simulink model "sampleModel1674_5_sub"  (R2023a)
settings: Solver=VariableStepAuto  StartTime=0.0  StopTime=10.0  RelTol=1e-3
libraries: hdlsllib x6, simulink x4
settings Model: Creator=user1  LastModifiedBy=user1

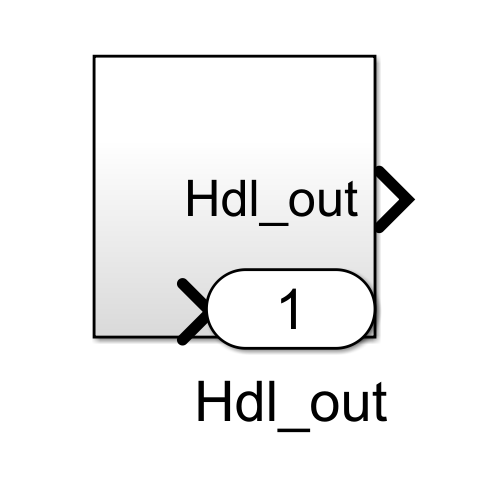
[thumbnail: Simulink's stored preview of the top-level diagram]
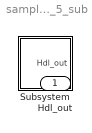
== system sampleModel1674_5_sub ==
  Subsystem : Subsystem
  Hdl_out : Outport  OutDataTypeStr=uint8

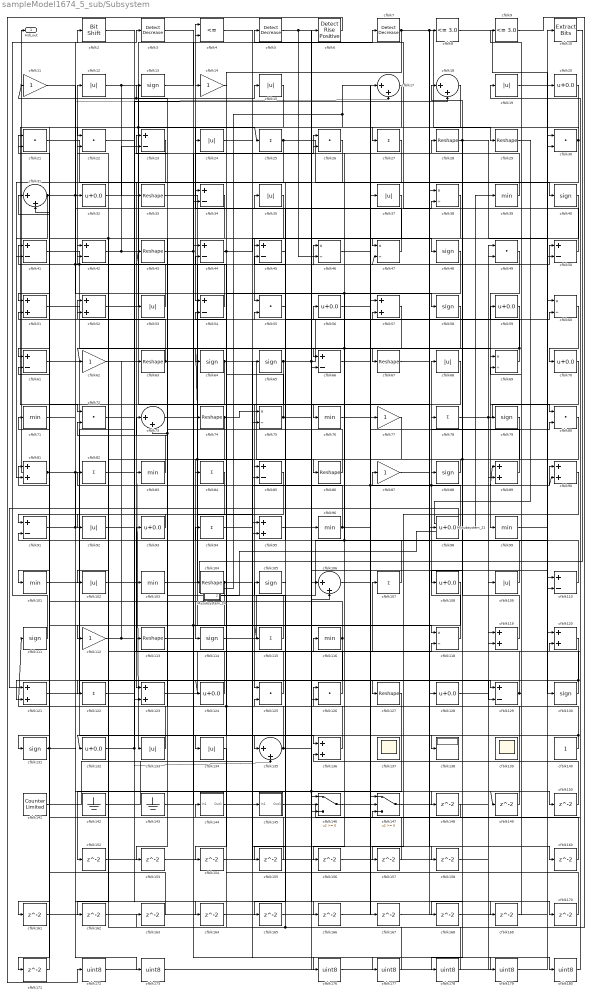
== system sampleModel1674_5_sub/Subsystem ==
  Mysubsystem_21 : Subsystem  TreatAsAtomicUnit=on  RTWFcnName=Mysubsystem_21
      settings: RTWFcnNameOpts=User specified  RTWFileNameOpts=Use function name
  Mysubsystem_24 : Subsystem  TreatAsAtomicUnit=on  RTWFcnName=Mysubsystem_24
      settings: RTWFcnNameOpts=User specified  RTWFileNameOpts=Use function name
  cfblk10 : simulink/Logic and Bit Operations/Extract Bits  bitsToExtract=Upper half  numBits=8  bitIdxRange=[0 7]  outScalingMode=Preserve fixed-point scaling
      settings: LibrarySourceBlock=|
      | hdlsllib/Logic and Bit
      | Operations/Extract Bits
  cfblk{39,71,76,83,96,99,101,103,116} (9 alike) : MinMax  OutDataTypeStr=uint8
  cfblk{12,15,19,24,35,37,53,68,92,102,109,133..134} (13 alike) : Abs  OutDataTypeStr=uint8  SaturateOnIntegerOverflow=off
  cfblk{28..29,33,43,63,67,74,86,104,113,127} (11 alike) : Reshape
  cfblk{13,40,48,58,64..65,79,88,105,111,114,130..131} (13 alike) : Signum
  cfblk{17..18,31,73,106,135} (6 alike) : Sum  Inputs=|++  OutDataTypeStr=uint8
  cfblk{25,27,78,82,84,94,107,115,122} (9 alike) : Sum  Inputs=+  OutDataTypeStr=uint8
  cfblk{20,32,56,59,70,93,98,108,124,128,132} (11 alike) : Bias  Bias=0.0  SaturateOnIntegerOverflow=off
  cfblk{11,14,62,77,87,112} (6 alike) : Gain  OutDataTypeStr=uint8
  cfblk{23,34,41..42,44..45,50,54,61,66,85,91,110,129} (14 alike) : Sum  Inputs=+-  OutDataTypeStr=uint8
  cfblk{38,46..47,60,69,75,118} (7 alike) : Product  Inputs=*/  OutDataTypeStr=uint8  RndMeth=Zero  SaturateOnIntegerOverflow=on
  cfblk{51..52,57,81,89..90,95,119..121,123,136} (12 alike) : Sum  OutDataTypeStr=uint8
  cfblk{21..22,26,30,49,55,72,80,125..126} (10 alike) : DotProduct  OutDataTypeStr=uint8
  cfblk137 : Scope
      settings: Floating=on
  cfblk138 : Display
  cfblk139 : Scope
      settings: Floating=on
  cfblk140 : Constant  OutDataTypeStr=uint8  SampleTime=-1
  cfblk141 : hdlsllib/Sources/Counter Limited  uplimit=7  tsamp=-1
  cfblk142 : Ground
  cfblk143 : Ground
  cfblk144 : Subsystem
      settings: LibrarySourceBlock=|
      | hdlsllib/Ports &
      | Subsystems/Subsystem
  cfblk145 : Subsystem
      settings: LibrarySourceBlock=|
      | hdlsllib/Ports &
      | Subsystems/Subsystem
  cfblk146 : Switch  OutDataTypeStr=uint8  SaturateOnIntegerOverflow=off  InputSameDT=off
  cfblk147 : Switch  OutDataTypeStr=uint8  SaturateOnIntegerOverflow=off  InputSameDT=off
  cfblk{148..150,152..158,160..171} (22 alike) : Delay  SampleTime=1
  cfblk{172..173,176..180} (7 alike) : DataTypeConversion  OutDataTypeStr=uint8  SaturateOnIntegerOverflow=off  RndMeth=Floor
  cfblk2 : hdlsllib/Logic and Bit Operations/Bit Shift  mode=Shift Left Logical  N=0
  cfblk3 : simulink/Logic and Bit Operations/Detect Decrease  vinit=0.0  OutDataTypeStr=uint8
      settings: LibrarySourceBlock=|
      | hdlsllib/Logic and Bit
      | Operations/Detect
      | Decrease
  cfblk4 : RelationalOperator  Operator=<=  OutDataTypeStr=boolean  InputSameDT=off
  cfblk5 : simulink/Logic and Bit Operations/Detect Decrease  vinit=0.0  OutDataTypeStr=uint8
      settings: LibrarySourceBlock=|
      | hdlsllib/Logic and Bit
      | Operations/Detect
      | Decrease
  cfblk6 : hdlsllib/Logic and Bit Operations/Detect Rise Positive  vinit=0  OutDataTypeStr=uint8
  cfblk7 : simulink/Logic and Bit Operations/Detect Decrease  vinit=0.0  OutDataTypeStr=uint8
      settings: LibrarySourceBlock=|
      | hdlsllib/Logic and Bit
      | Operations/Detect
      | Decrease
  cfblk8 : hdlsllib/Logic and Bit Operations/Compare To Constant  relop=<=  const=3.0  OutDataTypeStr=uint8
  cfblk9 : hdlsllib/Logic and Bit Operations/Compare To Constant  relop=<=  const=3.0  OutDataTypeStr=uint8
  Hdl_out : Outport  OutDataTypeStr=uint8
  wires:
  cfblk98/1 -> cfblk39/1, cfblk87/1
  cfblk34/1 -> cfblk162/1, cfblk161/1
  cfblk61/1 -> cfblk136/1
  cfblk7/1 -> cfblk34/1, cfblk160/1, cfblk29/1
  cfblk17/1 -> cfblk72/1
  cfblk50/1 -> cfblk5/1
  cfblk140/1 -> cfblk132/1, cfblk126/1
  cfblk43/1 -> cfblk179/1, cfblk26/2
  cfblk68/1 -> cfblk125/1
  cfblk74/1 -> cfblk75/1, cfblk114/1
  cfblk35/1 -> cfblk55/1
  cfblk101/1 -> cfblk129/1
  cfblk51/1 -> cfblk55/2
  cfblk120/1 -> cfblk178/1
  cfblk93/1 -> cfblk91/1
  cfblk3/1 -> cfblk177/1, cfblk115/1
  cfblk53/1 -> cfblk12/1
  cfblk30/1 -> cfblk27/1, cfblk85/1
  cfblk15/1 -> cfblk51/1
  cfblk79/1 -> cfblk168/1, cfblk133/1
  cfblk41/1 -> cfblk43/1, cfblk67/1
  cfblk145/1(Out1) -> cfblk19/1
  cfblk33/1 -> cfblk118/1
  cfblk71/1 -> cfblk17/2, cfblk32/1
  cfblk88/1 -> cfblk86/1
  cfblk125/1 -> cfblk42/1
  cfblk27/1 -> cfblk123/1
  cfblk11/1 -> cfblk58/1
  cfblk131/1 -> cfblk169/1, cfblk41/1
  cfblk94/1 -> cfblk149/1, cfblk146/3
  cfblk128/1 -> cfblk119/1
  cfblk64/1 -> cfblk101/1, cfblk96/1
  cfblk39/1 -> cfblk4/1
  cfblk67/1 -> cfblk8/1
  cfblk69/1 -> cfblk45/2, cfblk62/1
  cfblk47/1 -> cfblk14/1
  cfblk20/1 -> cfblk22/1
  cfblk42/1 -> cfblk23/2, cfblk4/2
  cfblk14/1 -> cfblk134/1
  cfblk65/1 -> cfblk113/1, cfblk110/2, cfblk57/2
  cfblk121/1 -> cfblk56/1
  cfblk126/1 -> cfblk93/1
  cfblk123/1 -> cfblk65/1
  cfblk8/1 -> cfblk110/1
  cfblk38/1 -> cfblk83/1, cfblk73/2
  cfblk76/1 -> cfblk17/1
  cfblk118/1 -> cfblk68/1
  cfblk83/1 -> cfblk72/2
  cfblk103/1 -> cfblk46/1
  cfblk73/1 -> cfblk145/1(In1), cfblk95/2
  cfblk129/1 -> cfblk82/1, cfblk9/1
  cfblk78/1 -> cfblk60/2, cfblk80/1
  cfblk119/1 -> cfblk18/1
  cfblk32/1 -> cfblk66/1
  cfblk85/1 -> cfblk123/2
  cfblk23/1 -> cfblk41/2
  cfblk12/1 -> cfblk33/1, cfblk25/1, cfblk147/2
  cfblk58/1 -> cfblk92/1
  cfblk4/1 -> cfblk48/1
  cfblk52/1 -> cfblk15/1
  cfblk107/1 -> cfblk26/1, cfblk81/1
  cfblk54/1 -> cfblk21/1
  cfblk111/1 -> cfblk2/1
  cfblk57/1 -> cfblk74/1, cfblk76/1
  cfblk136/1 -> cfblk94/1, cfblk111/1
  cfblk18/1 -> cfblk54/1
  cfblk87/1 -> cfblk128/1
  cfblk44/1 -> cfblk47/1, cfblk84/1
  cfblk25/1 -> cfblk40/1, cfblk131/1
  cfblk31/1 -> cfblk3/1, cfblk81/2
  cfblk60/1 -> cfblk70/1
  cfblk96/1 -> cfblk52/1, cfblk88/1, cfblk90/2
  cfblk112/1 -> cfblk63/1, cfblk53/1
  cfblk70/1 -> cfblk99/1
  cfblk130/1 -> cfblk124/1, cfblk107/1
  cfblk21/1 -> cfblk126/2
  cfblk147/1 -> cfblk49/1
  cfblk13/1 -> cfblk7/1
  cfblk114/1 -> cfblk10/1
  cfblk106/1 -> cfblk37/1
  cfblk116/1 -> cfblk51/2, cfblk121/2
  cfblk2/1 -> cfblk103/1
  cfblk46/1 -> cfblk77/1
  cfblk81/1 -> Hdl_out/1, cfblk146/2, cfblk50/1
  cfblk63/1 -> cfblk75/2, cfblk31/2
  cfblk89/1 -> cfblk78/1
  cfblk115/1 -> cfblk23/1
  cfblk99/1 -> cfblk30/2
  cfblk92/1 -> cfblk24/1
  cfblk40/1 -> cfblk61/1
  cfblk146/1 -> cfblk80/2, cfblk89/1
  cfblk75/1 -> cfblk44/2, cfblk127/1
  cfblk19/1 -> cfblk130/1
  cfblk141/1 -> cfblk44/1
  cfblk143/1 -> cfblk104/1
  cfblk49/1 -> cfblk79/1
  cfblk132/1 -> cfblk135/2, cfblk116/1
  cfblk109/1 -> cfblk28/1
  cfblk135/1 -> cfblk71/1, cfblk59/1
  cfblk91/1 -> cfblk173/1, cfblk47/2, cfblk38/2
  cfblk77/1 -> cfblk102/1
  cfblk86/1 -> cfblk13/1, cfblk11/1
  cfblk59/1 -> cfblk66/2
  cfblk104/1 -> cfblk180/1, cfblk122/1
  cfblk122/1 -> cfblk18/2
  cfblk95/1 -> cfblk106/2
  cfblk62/1 -> cfblk98/1
  cfblk124/1 -> cfblk52/2
  cfblk56/1 -> cfblk69/1
  cfblk37/1 -> cfblk112/1
  cfblk110/1 -> cfblk35/1
  cfblk5/1 -> cfblk170/1, cfblk46/2
  cfblk133/1 -> cfblk61/2
  cfblk28/1 -> cfblk50/2, cfblk108/1
  cfblk45/1 -> cfblk135/1
  cfblk113/1 -> cfblk118/2
  cfblk80/1 -> cfblk138/1
  cfblk48/1 -> cfblk156/1, cfblk64/1
  cfblk142/1 -> cfblk90/1
  cfblk26/1 -> cfblk45/1
  cfblk102/1 -> cfblk148/1
  cfblk148/1 -> cfblk147/3
  cfblk149/1 -> cfblk73/1
  cfblk72/1 -> cfblk150/1
  cfblk150/1 -> cfblk136/2
  cfblk127/1 -> cfblk152/1
  cfblk152/1 -> cfblk95/1
  cfblk84/1 -> cfblk153/1
  cfblk153/1 -> cfblk57/1
  cfblk134/1 -> cfblk154/1
  cfblk154/1 -> cfblk85/2
  cfblk55/1 -> cfblk155/1
  cfblk155/1 -> cfblk21/2
  cfblk156/1 -> cfblk49/2
  cfblk90/1 -> cfblk157/1
  cfblk157/1 -> cfblk125/2
  cfblk24/1 -> cfblk158/1
  cfblk158/1 -> cfblk89/2
  cfblk160/1 -> cfblk42/2
  cfblk161/1 -> cfblk147/1
  cfblk162/1 -> cfblk146/1
  cfblk9/1 -> cfblk163/1
  cfblk163/1 -> cfblk91/2
  cfblk82/1 -> cfblk164/1
  cfblk164/1 -> cfblk30/1
  cfblk105/1 -> cfblk165/1
  cfblk165/1 -> cfblk106/1
  cfblk22/1 -> cfblk166/1
  cfblk166/1 -> cfblk60/1
  cfblk66/1 -> cfblk167/1
  cfblk167/1 -> cfblk38/1
  cfblk168/1 -> cfblk119/2
  cfblk169/1 -> cfblk69/2
  cfblk170/1 -> cfblk54/2
  cfblk108/1 -> cfblk171/1
  cfblk171/1 -> cfblk31/1
  cfblk6/1 -> cfblk172/1
  cfblk172/1 -> cfblk20/1
  cfblk173/1 -> cfblk6/1
  cfblk144/1(Out1) -> cfblk176/1
  cfblk176/1 -> cfblk109/1
  cfblk177/1 -> cfblk144/1(In1)
  cfblk178/1 -> cfblk105/1, cfblk22/2
  cfblk179/1 -> cfblk120/1
  cfblk180/1 -> cfblk120/2
  cfblk29/1 -> Mysubsystem_21/1(In1)
  Mysubsystem_21/1(Out1) -> cfblk121/1
  Mysubsystem_24/1(Out1) -> cfblk34/2, cfblk129/2
  cfblk10/1 -> Mysubsystem_24/1(In1)
  Mysubsystem_24/2(Out2) -> Mysubsystem_21/2(In2)

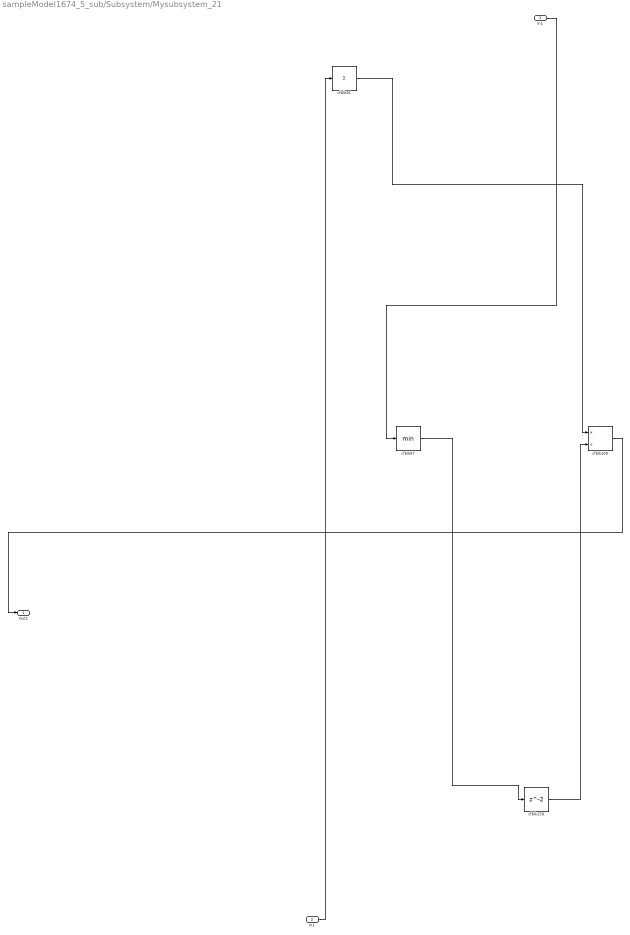
== system sampleModel1674_5_sub/Subsystem/Mysubsystem_21 ==
  In1 : Inport
  In2 : Inport  Port=2
  cfblk100 : Product  Inputs=*/  RndMeth=Zero  SaturateOnIntegerOverflow=on
  cfblk159 : Delay  SampleTime=1
  cfblk36 : Sum  Inputs=+
  cfblk97 : MinMax
  Out1 : Outport
  wires:
  In1/1 -> cfblk97/1
  cfblk100/1 -> Out1/1
  In2/1 -> cfblk36/1
  cfblk159/1 -> cfblk100/2
  cfblk36/1 -> cfblk100/1
  cfblk97/1 -> cfblk159/1

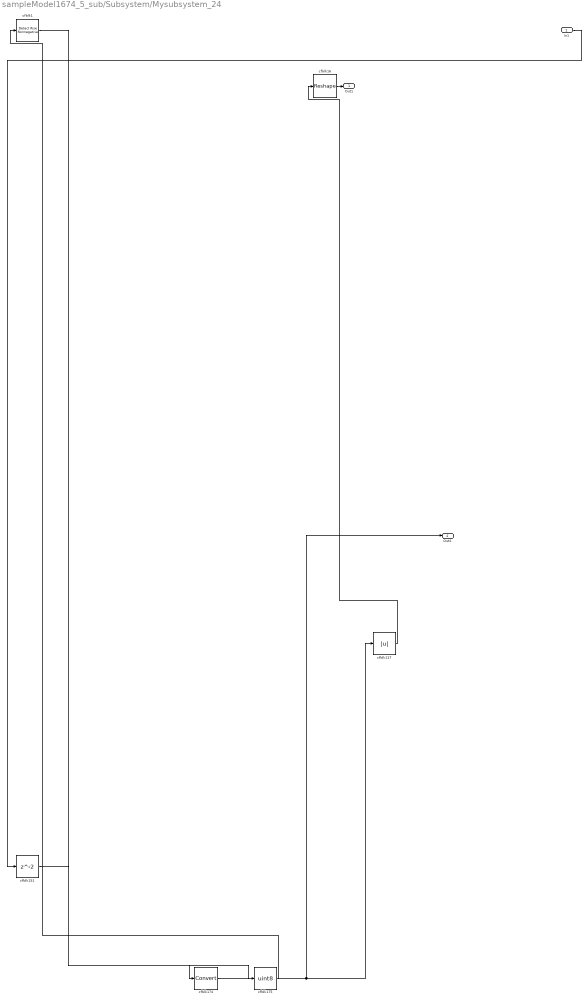
== system sampleModel1674_5_sub/Subsystem/Mysubsystem_24 ==
  In1 : Inport
  cfblk1 : hdlsllib/Logic and Bit Operations/Detect Rise Nonnegative  vinit=0  OutDataTypeStr=boolean
  cfblk117 : Abs  SaturateOnIntegerOverflow=off
  cfblk151 : Delay  SampleTime=1
  cfblk16 : Reshape
  cfblk174 : DataTypeConversion  SaturateOnIntegerOverflow=off  RndMeth=Floor
  cfblk175 : DataTypeConversion  OutDataTypeStr=uint8  SaturateOnIntegerOverflow=off  RndMeth=Floor
  Out1 : Outport
  Out2 : Outport  Port=2
  wires:
  cfblk151/1 -> cfblk175/1
  In1/1 -> cfblk151/1
  cfblk117/1 -> cfblk16/1
  cfblk1/1 -> cfblk174/1
  cfblk175/1 -> cfblk1/1
  cfblk16/1 -> Out1/1
  cfblk174/1 -> cfblk117/1, Out2/1

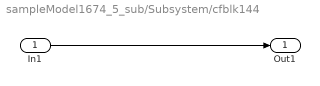
== system sampleModel1674_5_sub/Subsystem/cfblk144 ==
  In1 : Inport
  Out1 : Outport
  wires:
  In1/1 -> Out1/1

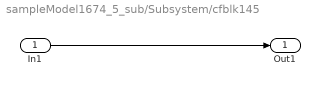
== system sampleModel1674_5_sub/Subsystem/cfblk145 ==
  In1 : Inport
  Out1 : Outport
  wires:
  In1/1 -> Out1/1
